simulink model "ReleaseQueue_Model"  (R2025a)
settings: Solver=VariableStepAuto  StartTime=0.0  StopTime=10.0  RelTol=1e-3
libraries: NSA_DEVS_LOGISTICS x9, NSA_DEVS_SINKS x6, NSA_DEVS_SOURCES x2
settings Model: Creator=peter  LastModifiedBy=peter

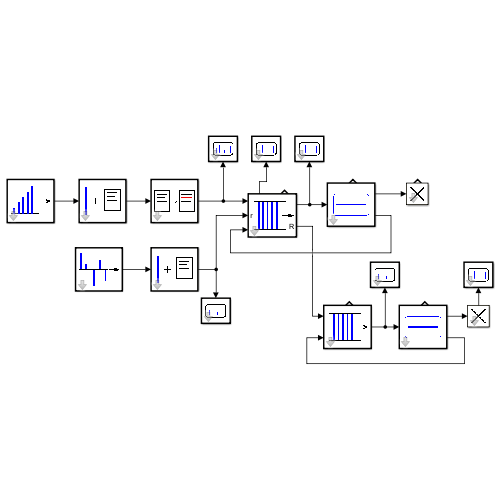
[thumbnail: Simulink's stored preview of the top-level diagram]
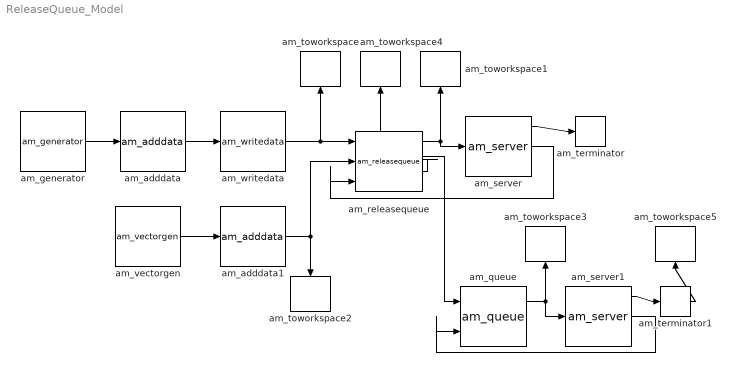
== system ReleaseQueue_Model ==
  am_adddata : NSA_DEVS_LOGISTICS/am_adddata  fields="\"value\""  values=[42]  numeric=[true]  infield="\"id\""  tau=[0,1]  debug=0
      settings: SourceProductName=Logistics
  am_adddata1 : NSA_DEVS_LOGISTICS/am_adddata  fields=[]  values=[]  numeric=[]  infield="\"value\""  tau=[0,1]  debug=0
      settings: SourceProductName=Logistics
  am_generator : NSA_DEVS_SOURCES/am_generator  tG=0.1  n0=1  nG=10  tD=[0,2]  debug=0
      settings: SourceProductName=Sources
  am_queue : NSA_DEVS_LOGISTICS/am_queue  tD=[0,2]  tau=[0,1]  debug=0
      settings: SourceProductName=Logistics
  am_releasequeue : NSA_DEVS_LOGISTICS/am_releasequeue  useSingleElementBatch=false  tD=[0,2]  tau=[0,1]  debug=0
      settings: SourceProductName=Logistics
  am_server : NSA_DEVS_LOGISTICS/am_server  tS=1.0  tsField="\"\""  tau=[0,1]  debug=0
      settings: SourceProductName=Logistics
  am_server1 : NSA_DEVS_LOGISTICS/am_server  tS=0.5  tsField="\"\""  tau=[0,1]  debug=0
      settings: SourceProductName=Logistics
  am_terminator : NSA_DEVS_LOGISTICS/am_terminator  tau=[0,1]  debug=0
      settings: SourceProductName=Logistics
  am_terminator1 : NSA_DEVS_LOGISTICS/am_terminator  tau=[0,1]  debug=0
      settings: SourceProductName=Logistics
  am_toworkspace : NSA_DEVS_SINKS/am_toworkspace  varname="\"in\""  t0=0  format="\"vector\""  tau=[0,5]  debug=0
      settings: SourceProductName=Sinks
  am_toworkspace1 : NSA_DEVS_SINKS/am_toworkspace  varname="\"out\""  t0=0  format="\"vector\""  tau=[0,5]  debug=0
      settings: SourceProductName=Sinks
  am_toworkspace2 : NSA_DEVS_SINKS/am_toworkspace  varname="\"rel\""  t0=0  format="\"vector\""  tau=[0,5]  debug=0
      settings: SourceProductName=Sinks
  am_toworkspace3 : NSA_DEVS_SINKS/am_toworkspace  varname="\"outR\""  t0=0  format="\"vector\""  tau=[0,5]  debug=0
      settings: SourceProductName=Sinks
  am_toworkspace4 : NSA_DEVS_SINKS/am_toworkspace  varname="\"nq\""  t0=0  format="\"vector\""  tau=[0,5]  debug=0
      settings: SourceProductName=Sinks
  am_toworkspace5 : NSA_DEVS_SINKS/am_toworkspace  varname="\"term\""  t0=0  format="\"vector\""  tau=[0,5]  debug=0
      settings: SourceProductName=Sinks
  am_vectorgen : NSA_DEVS_SOURCES/am_vectorgen  tvec=[2.5 100]  yvec=[1 42]  tau=[0,1]  debug=0
      settings: SourceProductName=Sources
  am_writedata : NSA_DEVS_LOGISTICS/am_writedata  inFields=[]  outField="\"value\""  changeFunc="\"out = randi(3);\""  tau=[0,1]  debug=0
      settings: SourceProductName=Logistics
  wires:
  am_generator/1 -> am_adddata/1
  am_adddata/1 -> am_writedata/1
  am_writedata/1 -> am_releasequeue/1, am_toworkspace/1
  am_server/2 -> am_releasequeue/3
  am_server/1 -> am_terminator/1
  am_vectorgen/1 -> am_adddata1/1
  am_adddata1/1 -> am_releasequeue/2, am_toworkspace2/1
  am_server1/1 -> am_terminator1/1
  am_queue/1 -> am_toworkspace3/1, am_server1/1
  am_server1/2 -> am_queue/2
  am_releasequeue/2 -> am_queue/1
  am_releasequeue/1 -> am_toworkspace1/1, am_server/1
  am_releasequeue/3 -> am_toworkspace4/1
  am_terminator1/1 -> am_toworkspace5/1
